simulink model "pid_func_simu"  (R2013a)
settings: Solver=ode45  StartTime=0.0  StopTime=10.0  RelTol=1e-3
undefined symbols (not defined in the file or in its folder): G1d
settings Model: Creator=mainster  LastModifiedBy=mainster

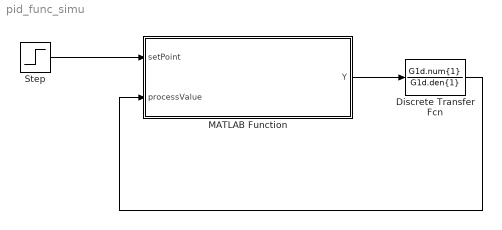
== system pid_func_simu ==
  Discrete Transfer Fcn : DiscreteTransferFcn  Numerator=G1d.num{1}  Denominator=G1d.den{1}  SampleTime=G1d.Ts
  MATLAB Function : MATLAB Function  TreatAsAtomicUnit=on
  Step : Step  SampleTime=0
  wires:
  MATLAB Function/1(Y) -> Discrete Transfer Fcn/1
  Discrete Transfer Fcn/1 -> MATLAB Function/2(processValue)
  Step/1 -> MATLAB Function/1(setPoint)

== matlab function pid_func_simu/MATLAB Function ==
  data: setPoint input; Y output; processValue input
function Y = fcn(setPoint, processValue)
%#codegen
Kp = 1.84;
Ki = 4.84e+03;
Kd = 0.000123;
Tf = 6.13e-05;
Ts = 5e-05;
%LE=length(time);
LE=35;

    yi=zeros(1,LE);
    yd=zeros(1,LE);
    Y=zeros(1,LE);
    e=zeros(1,LE);

    e(1) = setPoint(1) - processValue(1);
    yi(1) = Ki*Ts*e(1) - 0;
    yd(1) = (Kd * (e(1) - 0) + Tf * 0) / (Tf + Ts);
    Y(1) = Kp + yi(1) + yd(1);

    for k=2:LE
        e(k) = setPoint(k) - processValue(k);
        yi(k) = Ki*Ts*e(k) - yi(k-1);
        yd(k) = (Kd * (e(k) - e(k-1)) + Tf * yd(k-1)) / (Tf + Ts);
        Y(k) = Kp + yi(k) + yd(k);
    end

end
